simulink model "untitled"  (R2019a)
settings: Solver=VariableStepAuto  StartTime=0.0  StopTime=10.0  RelTol=1e-3
values from neighbouring files (symbols this model uses):
  g = 9.81    [pid_parameters.m]    (also in sample_file.m)
  I = 0.0068    [pid_parameters.m]    (also in sample_file.m = 0.05)
  Kd = -5    [pid_parameters.m]
  Ki = -5    [pid_parameters.m]
  Kp = -20    [pid_parameters.m]
  l = 0.4    [pid_parameters.m]    (also in sample_file.m = 0.3)
  M = 0.6    [pid_parameters.m]    (also in sample_file.m = 0.5)
  m = 0.09    [pid_parameters.m]    (also in sample_file.m = 0.2)
settings Model: Creator=robot  LastModifiedBy=robot

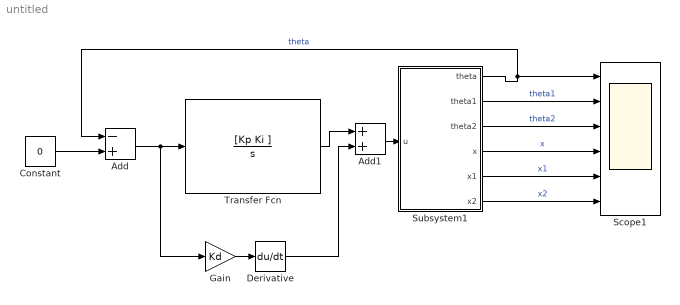
== system untitled ==
  Add : Sum  Inputs=-+
  Add1 : Sum
  Constant : Constant  Value=0
  Derivative : Derivative
  Gain : Gain  Gain=Kd
  Scope1 : Scope  NumInputPorts=6
  Subsystem1 : Subsystem
  Transfer Fcn : TransferFcn  Numerator=[Kp Ki ]  Denominator=[ 1 0]
  wires:
  Constant/1 -> Add/2
  Subsystem1/1(theta) -> Add/1, Scope1/1  "theta"
  Subsystem1/2(theta1) -> Scope1/2  "theta1"
  Subsystem1/3(theta2) -> Scope1/3  "theta2"
  Subsystem1/4(x) -> Scope1/4  "x"
  Subsystem1/5(x1) -> Scope1/5  "x1"
  Subsystem1/6(x2) -> Scope1/6  "x2"
  Add/1 -> Gain/1, Transfer Fcn/1
  Gain/1 -> Derivative/1
  Derivative/1 -> Add1/2
  Transfer Fcn/1 -> Add1/1
  Add1/1 -> Subsystem1/1(u)

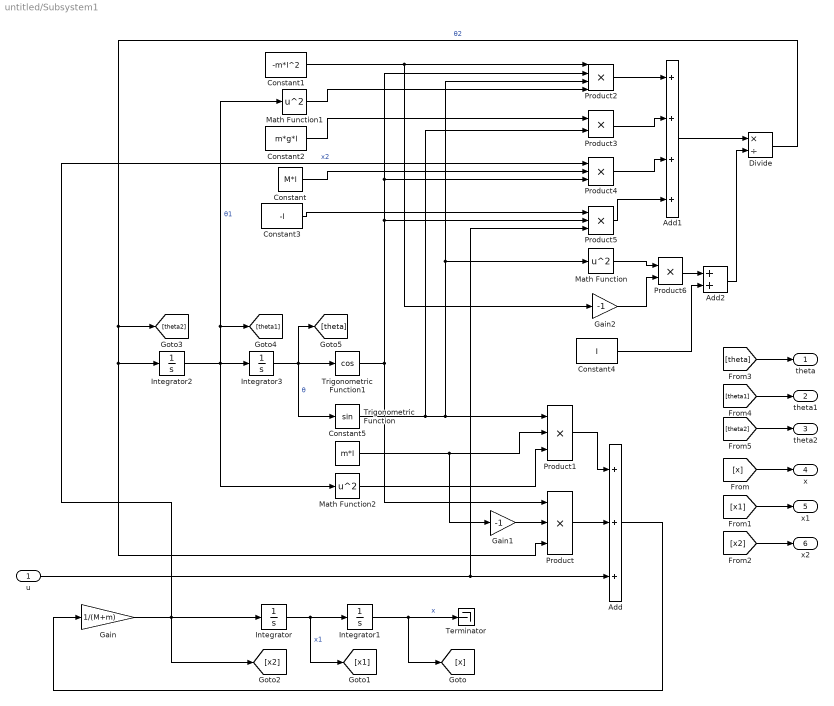
== system untitled/Subsystem1 ==
  u : Inport
  Add : Sum  Inputs=+++
  Add1 : Sum  Inputs=++++
  Add2 : Sum
  Constant : Constant  Value=M*l
  Constant1 : Constant  Value=-m*l^2
  Constant2 : Constant  Value=m*g*l
  Constant3 : Constant  Value=-l
  Constant4 : Constant  Value=I
  Constant5 : Constant  Value=m*l
  Divide : Product  Inputs=*/
  Gain : Gain  Gain=1/(M+m)
  Gain1 : Gain  Gain=-1
  Gain2 : Gain  Gain=-1
  Integrator : Integrator
  Integrator1 : Integrator
  Integrator2 : Integrator
  Integrator3 : Integrator  InitialCondition=1
  Math Function : Math  Operator=square  SaturateOnIntegerOverflow=on
  Math Function1 : Math  Operator=square  SaturateOnIntegerOverflow=on
  Math Function2 : Math  Operator=square  SaturateOnIntegerOverflow=on
  Product{,1,4..5} (4 alike) : Product  Inputs=3  RndMeth=Zero
  Product2 : Product  Inputs=4  RndMeth=Zero
  Product3 : Product  RndMeth=Zero
  Product6 : Product  RndMeth=Zero
  Terminator : Terminator
  Trigonometric Function : Trigonometry
  Trigonometric Function1 : Trigonometry  Operator=cos
  theta : Outport
  theta1 : Outport  Port=2
  theta2 : Outport  Port=3
  x : Outport  Port=4
  x1 : Outport  Port=5
  x2 : Outport  Port=6
  wires:
  [x] -> x/1
  [x1] -> x1/1
  [x2] -> x2/1
  [theta] -> theta/1
  [theta1] -> theta1/1
  [theta2] -> theta2/1
  Integrator1/1 -> Terminator/1, [x]  "x"
  Add/1 -> Gain/1
  u/1 -> Product5/3, Add/3
  Add1/1 -> Divide/1
  Add2/1 -> Divide/2
  Constant4/1 -> Add2/2
  Product6/1 -> Add2/1
  Math Function/1 -> Product6/1
  Product5/1 -> Add1/4
  Product4/1 -> Add1/3
  Product3/1 -> Add1/2
  Product2/1 -> Add1/1
  Constant3/1 -> Product5/1
  Constant2/1 -> Product3/1
  Constant1/1 -> Product2/1, Gain2/1
  Product1/1 -> Add/1
  Trigonometric Function1/1 -> Product2/2, Product4/3, Product5/2, Product/1
  Product/1 -> Add/2
  Constant/1 -> Product4/2
  Trigonometric Function/1 -> Product3/2, Product2/3, Math Function/1, Product1/1
  Integrator3/1 -> Trigonometric Function/1, Trigonometric Function1/1, [theta]  "θ"
  Integrator2/1 -> Integrator3/1, Math Function2/1, [theta1], Math Function1/1  "θ1"
  Divide/1 -> Integrator2/1, Product/3, [theta2]  "θ2"
  Integrator/1 -> Integrator1/1, [x1]  "x1"
  Gain/1 -> Integrator/1, [x2], Product4/1  "x2"
  Math Function1/1 -> Product2/4
  Gain2/1 -> Product6/2
  Gain1/1 -> Product/2
  Math Function2/1 -> Product1/3
  Constant5/1 -> Product1/2, Gain1/1
